simulink model "FAST_RL_Env"  (R2023a)
settings: Solver=FixedStepAuto  StartTime=0.0  StopTime=inf  FixedStep=DT  MaxStep=DT  RelTol=1e-3  EnableMultiTasking=on
values from neighbouring files (symbols this model uses):
  Cmoment = 3    [HyperparameterSearch_BN_LSTM.m]    (also in HyperparameterSearch_BatchSize.m = 2.5; HyperparameterSearch_LearningRate.m = 2.5; HyperparameterSearch_NeuronLayer.m = 2.5; RunFASTnet_train.m = 1)
  Cpitch = 0    [HyperparameterSearch_BN_LSTM.m]    (also in HyperparameterSearch_BatchSize.m = 0.5; HyperparameterSearch_LearningRate.m = 0.5; HyperparameterSearch_NeuronLayer.m = 0.5; RunFASTnet_train.m)
libraries: rllib x1
settings Model: Creator=bjonkman  LastModifiedBy=Admin
settings SolverCC: AlgebraicLoopSolver=TrustRegion  AutoInsertRateTranBlk=on
settings DataIOCC: LimitDataPoints=on  SaveFormat=Array  SignalLoggingSaveFormat=ModelDataLogs  SaveOutput=off  SaveTime=off  SignalLoggingName=sigsOut
settings OptimizationCC: ReuseModelBlockBuffer=off  ExpressionDepthLimit=2147483647  LifeSpan=inf
settings DebuggingCC: SaveWithParameterizedLinksMsg=none  UnderspecifiedInitializationDetection=Classic  MergeDetectMultiDrivingBlocksExec=none  SignalResolutionControl=TryResolveAllWithWarning  MultiTaskDSMMsg=warning  MultiTaskCondExecSysMsg=none  FcnCallInpInsideContextMsg=warning  UnconnectedInputMsg=warning  UnconnectedOutputMsg=warning  UnconnectedLineMsg=warning  StateNameClashWarn=warning  SFUnexpectedBacktrackingDiag=warning  SFNoUnconditionalDefaultTransitionDiag=warning  SFExecutionAtInitializationDiag=none  ArithmeticOperatorsInVariantConditions=warning
settings HardwareCC: ProdBitPerPointer=32  ProdBitPerSizeT=32  ProdBitPerPtrDiffT=32  ProdLargestAtomicFloat=None  ProdIntDivRoundTo=Undefined  ProdEndianess=Unspecified  ProdWordSize=32  ProdHWDeviceType=32-bit Generic  TargetUnknown=on
settings ModelReferenceCC: EnableRefExpFcnMdlSchedulingChecks=on  PropagateSignalLabelsOutOfModel=off
settings SFSimCC: SimUseLocalCustomCode=off  CustomCodeUndefinedFunction=UseInterfaceOnly
settings RTWCC: RTWUseLocalCustomCode=off  DLArmComputeVersion=19.05
settings CodeAppCC: StateflowObjectComments=on
settings GRTTargetCC: TargetLangStandard=C89/C90 (ANSI)  CombineOutputUpdateFcns=off  GRTInterface=on
settings ConfigComp: CovMetricSettings=dw  CovSaveCumulativeToWorkspaceVar=on  CovSaveSingleToWorkspaceVar=on  CovExternalEMLEnable=off

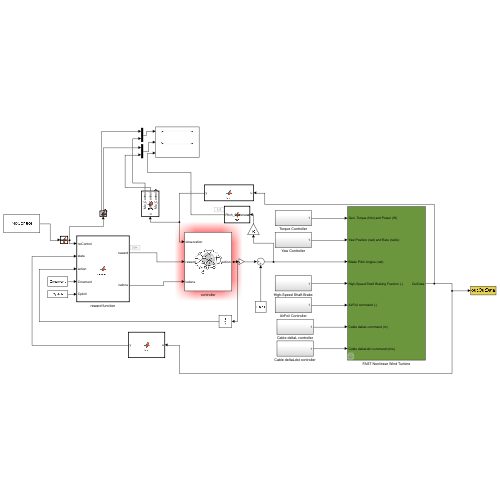
[thumbnail: Simulink's stored preview of the top-level diagram]
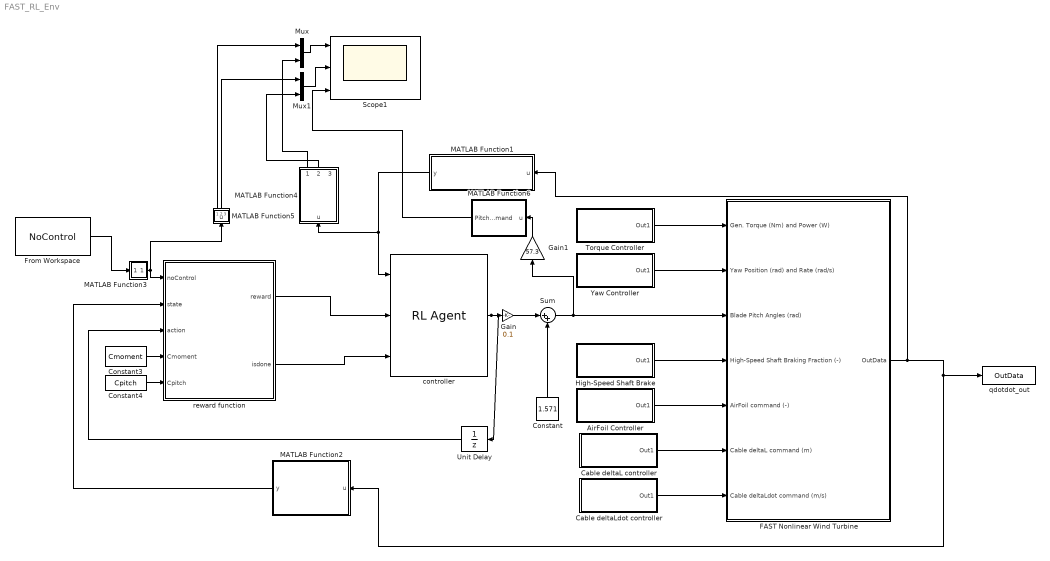
== system FAST_RL_Env ==
  AirFoil Controller : Subsystem
  Cable deltaL controller : Subsystem
  Cable deltaLdot controller : Subsystem
  Constant : Constant  Value=1.571
  Constant3 : Constant  Value=Cmoment
  Constant4 : Constant  Value=Cpitch
  FAST Nonlinear Wind Turbine : Subsystem  mask(FAST Nonlinear Wind Turbine){}
      mask help: This block contains the FAST S-Function.
      mask init:
      | clear FAST_SFunc
  From Workspace : FromWorkspace  VariableName=NoControl
  Gain : Gain  Gain=0.1
  Gain1 : Gain  Gain=57.3
  High-Speed Shaft Brake : Subsystem
  MATLAB Function1 : MATLAB Function  TreatAsAtomicUnit=on
  MATLAB Function2 : MATLAB Function  TreatAsAtomicUnit=on
  MATLAB Function3 : MATLAB Function  TreatAsAtomicUnit=on
  MATLAB Function4 : MATLAB Function  TreatAsAtomicUnit=on
  MATLAB Function5 : MATLAB Function  TreatAsAtomicUnit=on
  MATLAB Function6 : MATLAB Function  TreatAsAtomicUnit=on
  Mux : Mux  Inputs=2
  Mux1 : Mux  Inputs=2
  Scope1 : Scope  NumInputPorts=3
  Sum : Sum  Inputs=|++
  Torque Controller : Subsystem
  Unit Delay : UnitDelay  SampleTime=-1  HasFrameUpgradeWarning=on
  Yaw Controller : Subsystem
  controller : rllib/RL Agent  Agent=agent  ExternalActionAsInput=off  ProvideLastAction=off  ProvideCumRwd=off  TreatAsDirectFeedthrough=on  UseStrictObservationDataTypes=off
  qdotdot_out : ToWorkspace  VariableName=OutData  SampleTime=-1
  reward function : MATLAB Function  TreatAsAtomicUnit=on
  wires:
  Torque Controller/1(Out1) -> FAST Nonlinear Wind Turbine/1(Gen. Torque (Nm) and Power (W))
  Yaw Controller/1(Out1) -> FAST Nonlinear Wind Turbine/2(Yaw Position (rad) and Rate (rad/s))
  High-Speed Shaft Brake/1(Out1) -> FAST Nonlinear Wind Turbine/4(High-Speed Shaft Braking Fraction (-))
  AirFoil Controller/1(Out1) -> FAST Nonlinear Wind Turbine/5(AirFoil command (-))
  reward function/1(reward) -> controller/2
  Unit Delay/1 -> reward function/3(action)
  Cable deltaL controller/1(Out1) -> FAST Nonlinear Wind Turbine/6(Cable deltaL command (m))
  Cable deltaLdot controller/1(Out1) -> FAST Nonlinear Wind Turbine/7(Cable deltaLdot command (m/s))
  FAST Nonlinear Wind Turbine/1(OutData) -> MATLAB Function1/1(u), qdotdot_out/1, MATLAB Function2/1(u)
  MATLAB Function2/1(y) -> reward function/2(state)
  MATLAB Function1/1(y) -> MATLAB Function4/1(u), controller/1
  Constant4/1 -> reward function/5(Cpitch)
  Constant3/1 -> reward function/4(Cmoment)
  controller/1 -> Unit Delay/1, Gain/1
  reward function/2(isdone) -> controller/3
  From Workspace/1 -> MATLAB Function3/1(u)
  MATLAB Function3/1(NoControlMoments) -> reward function/1(noControl), MATLAB Function5/1(u)
  MATLAB Function5/1(Mx_No_Control) -> Mux/1
  MATLAB Function5/2(My_No_Control) -> Mux1/1
  MATLAB Function4/1(Mx_Control) -> Mux/2
  MATLAB Function4/2(My_Control) -> Mux1/2
  Mux/1 -> Scope1/1
  Mux1/1 -> Scope1/2
  Gain1/1 -> MATLAB Function6/1(u)
  MATLAB Function6/1(Pitch_Command) -> Scope1/3
  Constant/1 -> Sum/2
  Gain/1 -> Sum/1
  Sum/1 -> FAST Nonlinear Wind Turbine/3(Blade Pitch Angles (rad)), Gain1/1

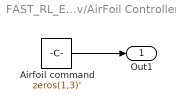
== system FAST_RL_Env/AirFoil Controller ==
  Airfoil command : Constant  Value=zeros(1,3)'
  Out1 : Outport
  wires:
  Airfoil command/1 -> Out1/1

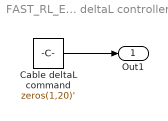
== system FAST_RL_Env/Cable deltaL controller ==
  Cable deltaL command : Constant  Value=zeros(1,20)'
  Out1 : Outport
  wires:
  Cable deltaL command/1 -> Out1/1

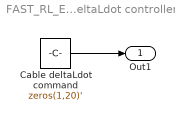
== system FAST_RL_Env/Cable deltaLdot controller ==
  Cable deltaLdot command : Constant  Value=zeros(1,20)'
  Out1 : Outport
  wires:
  Cable deltaLdot command/1 -> Out1/1

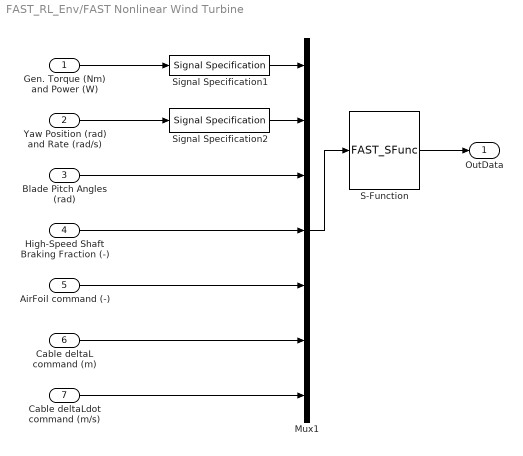
== system FAST_RL_Env/FAST Nonlinear Wind Turbine ==
  Gen. Torque (Nm) and Power (W) : Inport
  Yaw Position (rad) and Rate (rad/s) : Inport  Port=2
  Blade Pitch Angles (rad) : Inport  Port=3
  High-Speed Shaft Braking Fraction (-) : Inport  Port=4
  AirFoil command (-) : Inport  Port=5
  Cable deltaL command (m) : Inport  Port=6
  Cable deltaLdot command (m/s) : Inport  Port=7
  Mux1 : Mux  Inputs=7
  S-Function : S-Function  FunctionName=FAST_SFunc  Parameters=FAST_InputFileName, TMax, 0  SFunctionDeploymentMode=off  EnableBusSupport=off
  Signal Specification1 : SignalSpecification  OutDataTypeStr=double  Dimensions=2
  Signal Specification2 : SignalSpecification  OutDataTypeStr=double  Dimensions=2
  OutData : Outport
  wires:
  Gen. Torque (Nm) and Power (W)/1 -> Signal Specification1/1
  S-Function/1 -> OutData/1
  Mux1/1 -> S-Function/1
  Blade Pitch Angles (rad)/1 -> Mux1/3
  Yaw Position (rad) and Rate (rad/s)/1 -> Signal Specification2/1
  Signal Specification1/1 -> Mux1/1
  Signal Specification2/1 -> Mux1/2
  High-Speed Shaft Braking Fraction (-)/1 -> Mux1/4
  AirFoil command (-)/1 -> Mux1/5
  Cable deltaL command (m)/1 -> Mux1/6
  Cable deltaLdot command (m/s)/1 -> Mux1/7

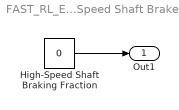
== system FAST_RL_Env/High-Speed Shaft Brake ==
  High-Speed Shaft Braking Fraction : Constant  Value=0
  Out1 : Outport
  wires:
  High-Speed Shaft Braking Fraction/1 -> Out1/1

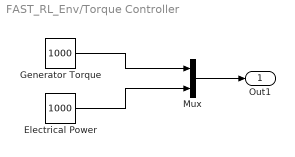
== system FAST_RL_Env/Torque Controller ==
  Electrical Power : Constant  Value=1000
  Generator Torque : Constant  Value=1000
  Mux : Mux  Inputs=2
  Out1 : Outport
  wires:
  Mux/1 -> Out1/1
  Generator Torque/1 -> Mux/1
  Electrical Power/1 -> Mux/2

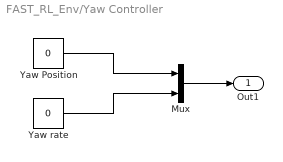
== system FAST_RL_Env/Yaw Controller ==
  Mux : Mux  Inputs=2
  Yaw Position : Constant  Value=0
  Yaw rate : Constant  Value=0
  Out1 : Outport
  wires:
  Mux/1 -> Out1/1
  Yaw Position/1 -> Mux/1
  Yaw rate/1 -> Mux/2

== matlab function FAST_RL_Env/reward function ==
  data: noControl input; state input; action input; reward output; Cmoment input; Cpitch input; isdone output
function [reward,isdone]   = reward(noControl,state, action, Cmoment,Cpitch)

%roll = state(18)/;
%pitch = state(16);
%surge = state(12);
%sway = state(16);
%heave = state(14);

%basemoment = state(36);
%power = state(39)/100000;
rollMoment = abs(state(1)) ;
pitchMoment = abs(state(2)) ;
yawMoment = abs(state(3)) ;

isdone = false ;
%moveLine1 = action(1);

reward = -Cmoment*((rollMoment)^2-abs(noControl(1))^2) - Cmoment*((pitchMoment)^2-abs(noControl(2))^2) ;
% if abs(rollMoment) > 1 || abs(pitchMoment) > 1 || abs(yawMoment) > 1 
%     isdone = true ;
%     reward = reward - Penalty ;
% else
%     isdone = false;
% end

== matlab function FAST_RL_Env/MATLAB Function1 ==
  data: u input; y output
function y  = fcn(u)

y = [u(39,:)/7.629e4, u(40,:)/5.8326e4, u(41,:)/1.3447e3,u(48,:),u(18,:),u(19,:)] ; %Heave

== matlab function FAST_RL_Env/MATLAB Function2 ==
  data: u input; y output
function y  = fcn(u)

y = [u(39,:)/7.629e4, u(40,:)/5.8326e4, u(41,:)/1.3447e3] ; %Heave

== matlab function FAST_RL_Env/MATLAB Function3 ==
  data: u input; NoControlMoments output
function NoControlMoments  = fcn(u)
% dt = 0.1 ;
%  i = 5001-time/dt ;
NoControlMoments = [u(1)/7.629e4 , u(2)/5.8326e4, u(3)/1.3447e3] ; %Heave

== matlab function FAST_RL_Env/MATLAB Function4 ==
  data: u input; Mx_Control output; My_Control output; Mz_Control output
function [Mx_Control,My_Control,Mz_Control] = fcn(u)

Mx_Control = u(2) ;
My_Control = u(3) ;
Mz_Control = u(4) ;

== matlab function FAST_RL_Env/MATLAB Function5 ==
  data: u input; Mx_No_Control output; My_No_Control output; Mz_No_Control output
function [Mx_No_Control,My_No_Control,Mz_No_Control] = fcn(u)

Mx_No_Control = u(1) ;
My_No_Control = u(2) ;
Mz_No_Control = u(3) ;

== matlab function FAST_RL_Env/MATLAB Function6 ==
  data: u input; Pitch_Command output
function Pitch_Command = fcn(u)

Pitch_Command = u;
